simulink model "engine_model_181218"  (R2018b)
settings: Solver=VariableStepAuto  StartTime=0.0  StopTime=20  FixedStep=0.001  RelTol=1e-3
values from neighbouring files (symbols this model uses):
  F = 5e-5    (= 5e-05)    [BLDC_simulator.m]    (also in engine_parameters.m; engine_parameters_20191210.m = 1)
  J = 7.22e-6    (= 7.22e-06)    [BLDC_simulator.m]    (also in IMU.m = [cos(theta_2)*cos(theta_3) sin(theta_3) 0; engine_parameters.m; engine_parameters_20191210.m = 0.001)
  Kt = 8.44e-3    (= 0.00844)    [BLDC_simulator.m]    (also in engine_parameters.m)
  Kv = 8.44e-3    (= 0.00844)    [BLDC_simulator.m]    (also in engine_parameters.m)
  L = 0.42e-3    (= 0.00042)    [BLDC_simulator.m]    (also in engine_parameters.m; engine_parameters_20191210.m = 0.0005)
  R = 7.9    [BLDC_simulator.m]    (also in engine_parameters.m; engine_parameters_20191210.m = 0.5; inversekinematics.m = Rg*Rd*Rm)
libraries: simulink x2
settings Model: Creator=Paweł Tymiński  LastModifiedBy=Paweł Tymiński

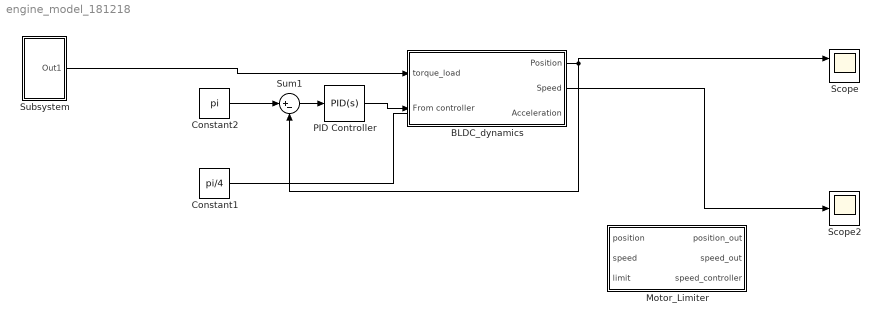
== system engine_model_181218 ==
  BLDC_dynamics : Subsystem
  Constant1 : Constant  Value=pi/4
  Constant2 : Constant  Value=pi
  Motor_Limiter : MATLAB Function  TreatAsAtomicUnit=on
  PID Controller : simulink/Continuous/PID Controller  Controller=PID  Form=Ideal  TimeDomain=Continuous-time  SampleTime=-1  IntegratorMethod=Forward Euler  FilterMethod=Forward Euler  ControllerParametersSource=internal  P=3.75221520248844  I=9.20583270553454  D=0.233305479962469  UseFilter=on  N=39454.8430256031  TunerSelectOption=Transfer Function Based (PID Tuner App)  InitialConditionSource=internal  InitialConditionForIntegrator=0  InitialConditionForFilter=0  DifferentiatorICPrevScaledInput=0  ExternalReset=none  TrackingMode=off  Kt=1  LimitOutput=off  UpperSaturationLimit=inf  LowerSaturationLimit=-inf  LinearizeAsGain=on  AntiWindupMode=none  Kb=1  POutMin=[]  POutMax=[]  IOutMin=[]  IOutMax=[]  DOutMin=[]  DOutMax=[]  NOutMin=[]  NOutMax=[]  SumOutMin=[]  SumOutMax=[]  SaturationOutMin=[]  SaturationOutMax=[]  PParamMin=[]  PParamMax=[]  IParamMin=[]  IParamMax=[]  DParamMin=[]  DParamMax=[]  NParamMin=[]  NParamMax=[]  KbParamMin=[]  KbParamMax=[]  KtParamMin=[]  KtParamMax=[]  KbOutMin=[]  KbOutMax=[]  KtOutMin=[]  KtOutMax=[]  IntegratorOutMin=[]  IntegratorOutMax=[]  FilterOutMin=[]  FilterOutMax=[]  SumI1OutMin=[]  SumI1OutMax=[]  SumI2OutMin=[]  SumI2OutMax=[]  SumI3OutMin=[]  SumI3OutMax=[]  SumI4OutMin=[]  SumI4OutMax=[]  SumDOutMin=[]  SumDOutMax=[]  DifferentiatorOutMin=[]  DifferentiatorOutMax=[]  FilterDiffOutCoefMin=[]  FilterDiffOutCoefMax=[]  ReciprocalOutMin=[]  ReciprocalOutMax=[]  SumDenOutMin=[]  SumDenOutMax=[]  SumNumOutMin=[]  SumNumOutMax=[]  DivideOutMin=[]  DivideOutMax=[]  IntegratorContinuousStateAttributes=''  IntegratorStateMustResolveToSignalObject=off  IntegratorRTWStateStorageClass=Auto  FilterContinuousStateAttributes=''  FilterStateMustResolveToSignalObject=off  FilterRTWStateStorageClass=Auto  ParallelPVariant=Passthrough  IdealPVariant=InternalParameters  IVariant=InternalParameters  DVariant=InternalParameters  IntegratorVariant=Continuous  SatVariant=Disabled  AWVariant=Passthrough  PCopyVariant=Disabled  TRVariant=Disabled  FdbkBlocksVariant=Forward  IdealPFdbkVariant=Disabled  SatFdbkVariant=Disabled  DerivativeFilterVariant=ContFilter  NVariant=InternalParameters  NCopyVariant=Disabled  FilterICVariant=InternalICsFilter  IntegratorICVariant=InternalICs  ExternalResetVariant=Disabled  TRSumVariant=Passthrough  SumFdbkVariant=Disabled  SumVariant=Sum_PID
  Scope : Scope  NumInputPorts=2
  Scope2 : Scope
  Subsystem : Subsystem
  Sum1 : Sum  Inputs=|+-
  wires:
  BLDC_dynamics/1(Position) -> Scope/1, Sum1/2
  PID Controller/1 -> BLDC_dynamics/2(From controller)
  Sum1/1 -> PID Controller/1
  Constant2/1 -> Sum1/1
  Subsystem/1(Out1) -> BLDC_dynamics/1(torque_load)
  Constant1/1 -> ?
  ? -> Scope/2
  BLDC_dynamics/2(Speed) -> Scope2/1

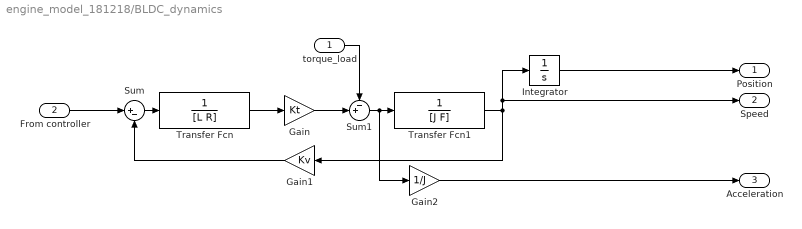
== system engine_model_181218/BLDC_dynamics ==
  torque_load : Inport
  From controller : Inport  Port=2
  Gain : Gain  Gain=Kt
  Gain1 : Gain  Gain=Kv
  Gain2 : Gain  Gain=1/J
  Integrator : Integrator
  Sum : Sum  Inputs=|+-
  Sum1 : Sum  Inputs=-+|
  Transfer Fcn : TransferFcn  Denominator=[L R]
  Transfer Fcn1 : TransferFcn  Denominator=[J F]
  Position : Outport
  Speed : Outport  Port=2
  Acceleration : Outport  Port=3
  wires:
  Gain/1 -> Sum1/2
  Transfer Fcn/1 -> Gain/1
  Sum/1 -> Transfer Fcn/1
  From controller/1 -> Sum/1
  torque_load/1 -> Sum1/1
  Gain1/1 -> Sum/2
  Sum1/1 -> Gain2/1, Transfer Fcn1/1
  Gain2/1 -> Acceleration/1
  Transfer Fcn1/1 -> Speed/1, Integrator/1, Gain1/1
  Integrator/1 -> Position/1

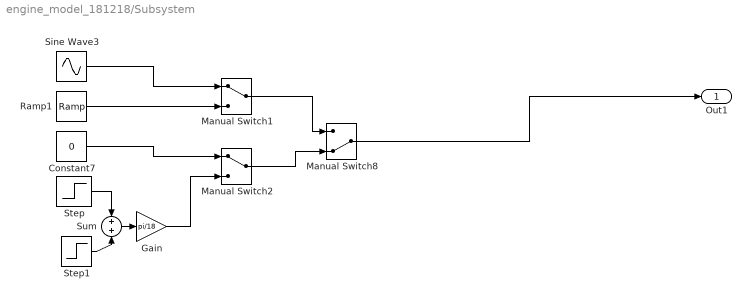
== system engine_model_181218/Subsystem ==
  Constant7 : Constant  Value=0
  Gain : Gain  Gain=pi/18
  Manual Switch1 : ManualSwitch
  Manual Switch2 : ManualSwitch
  Manual Switch8 : ManualSwitch  CurrentSetting=0
  Ramp1 : simulink/Sources/Ramp  slope=pi/16  start=0  InitialOutput=0
  Sine Wave3 : Sin  Amplitude=pi/18  SampleTime=0
  Step : Step  SampleTime=0
  Step1 : Step  Time=4  After=-1  SampleTime=0
  Sum : Sum
  Out1 : Outport
  wires:
  Step/1 -> Sum/1
  Constant7/1 -> Manual Switch2/1
  Gain/1 -> Manual Switch2/2
  Step1/1 -> Sum/2
  Sine Wave3/1 -> Manual Switch1/1
  Manual Switch1/1 -> Manual Switch8/1
  Manual Switch2/1 -> Manual Switch8/2
  Sum/1 -> Gain/1
  Ramp1/1 -> Manual Switch1/2
  Manual Switch8/1 -> Out1/1

== matlab function engine_model_181218/Motor_Limiter ==
  data: position input; position_out output; speed input; speed_out output; limit input; speed_controller output
function [position_out,speed_out, speed_controller] = fcn(position, speed, limit)
speed_controller=speed;
if abs(position)<limit        
    position_out=position;
    speed_out=speed;
else
    position_out=sign(position)*limit;   
    speed_out=0;
end
